simulink model "TesteMalhaExternaR2018b"  (R2018b)
settings: Solver=ode23s  StartTime=0.0  StopTime=10.0  RelTol=1e-3
values from neighbouring files (symbols this model uses):
  x = fmincon(@otimiza_PIDF,x,[],[],[],[],[0 0 0 0],[inf inf inf inf],@QQQ,options)    [Main_Malha_Externa.m]    (also in Main_Malha_Externa_referencia.m; main.m = fmincon(@otimiza_Esq,x,[],[],[],[],[0 0 0],[inf inf 1400],@Q; main_malha_interna.m = fmincon(@otimiza_Esq,x,[],[],[],[],[0 0 0],[inf inf 1400],@Q; otimiza_Dir.m = X)
libraries: simulink x1
settings Model: Creator=lucas  LastModifiedBy=vitor
settings DataIOCC: ReturnWorkspaceOutputs=on
settings DebuggingCC: SFMachineParentedDataDiag=error

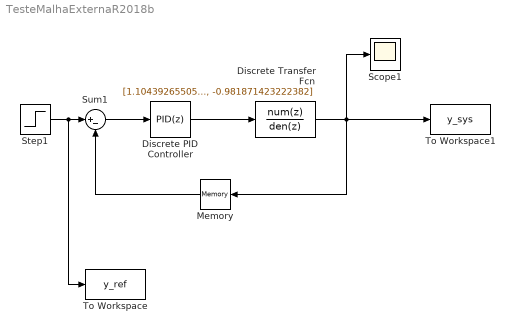
== system TesteMalhaExternaR2018b ==
  Discrete Transfer Fcn : DiscreteTransferFcn  Numerator=[1.104392655054829e-08, 3.313177965164485e-08, 3.313177965164485e-08, 1.104392655054829e-08]  Denominator=[1, -2.981694681338594, 2.963566104560976, -0.981871423222382]
  Discrete PID Controller : simulink/Continuous/PID Controller  Controller=PID  Form=Parallel  TimeDomain=Discrete-time  SampleTime=-1  IntegratorMethod=Forward Euler  FilterMethod=Forward Euler  ControllerParametersSource=internal  P=x(1)  I=x(2)  D=x(3)  UseFilter=on  N=x(4)  TunerSelectOption=Transfer Function Based (PID Tuner App)  InitialConditionSource=internal  InitialConditionForIntegrator=0  InitialConditionForFilter=0  DifferentiatorICPrevScaledInput=0  ExternalReset=none  TrackingMode=off  Kt=1  LimitOutput=off  UpperSaturationLimit=inf  LowerSaturationLimit=-inf  LinearizeAsGain=off  AntiWindupMode=none  Kb=1  POutMin=[]  POutMax=[]  IOutMin=[]  IOutMax=[]  DOutMin=[]  DOutMax=[]  NOutMin=[]  NOutMax=[]  SumOutMin=[]  SumOutMax=[]  SaturationOutMin=[]  SaturationOutMax=[]  PParamMin=[]  PParamMax=[]  IParamMin=[]  IParamMax=[]  DParamMin=[]  DParamMax=[]  NParamMin=[]  NParamMax=[]  KbParamMin=[]  KbParamMax=[]  KtParamMin=[]  KtParamMax=[]  KbOutMin=[]  KbOutMax=[]  KtOutMin=[]  KtOutMax=[]  IntegratorOutMin=[]  IntegratorOutMax=[]  FilterOutMin=[]  FilterOutMax=[]  SumI1OutMin=[]  SumI1OutMax=[]  SumI2OutMin=[]  SumI2OutMax=[]  SumI3OutMin=[]  SumI3OutMax=[]  SumI4OutMin=[]  SumI4OutMax=[]  SumDOutMin=[]  SumDOutMax=[]  DifferentiatorOutMin=[]  DifferentiatorOutMax=[]  FilterDiffOutCoefMin=[]  FilterDiffOutCoefMax=[]  ReciprocalOutMin=[]  ReciprocalOutMax=[]  SumDenOutMin=[]  SumDenOutMax=[]  SumNumOutMin=[]  SumNumOutMax=[]  DivideOutMin=[]  DivideOutMax=[]  IntegratorContinuousStateAttributes=''  IntegratorStateMustResolveToSignalObject=off  IntegratorRTWStateStorageClass=Auto  FilterContinuousStateAttributes=''  FilterStateMustResolveToSignalObject=off  FilterRTWStateStorageClass=Auto  ParallelPVariant=InternalParameters  IdealPVariant=Disabled  IVariant=InternalParameters  DVariant=InternalParameters  IntegratorVariant=Discrete  SatVariant=Disabled  AWVariant=Passthrough  PCopyVariant=Disabled  TRVariant=Disabled  FdbkBlocksVariant=Forward  IdealPFdbkVariant=Disabled  SatFdbkVariant=Disabled  DerivativeFilterVariant=ForwardEulerFilter  NVariant=InternalParameters  NCopyVariant=Disabled  FilterICVariant=InternalICsFilter  IntegratorICVariant=InternalICs  ExternalResetVariant=Disabled  TRSumVariant=Passthrough  SumFdbkVariant=Disabled  SumVariant=Sum_PID
  Memory : Memory  InheritSampleTime=on
  Scope1 : Scope
  Step1 : Step  Time=0  After=0.3  SampleTime=0.001
  Sum1 : Sum  Inputs=|+-
  To Workspace : ToWorkspace  VariableName=y_ref  SampleTime=-1
  To Workspace1 : ToWorkspace  VariableName=y_sys  SampleTime=-1
  wires:
  Step1/1 -> To Workspace/1, Sum1/1
  Sum1/1 -> Discrete PID Controller/1
  Discrete PID Controller/1 -> Discrete Transfer Fcn/1
  Discrete Transfer Fcn/1 -> To Workspace1/1, Memory/1, Scope1/1
  Memory/1 -> Sum1/2
